simulink model "compute_next_state_2019a"  (R2019a)
settings: Solver=FixedStepAuto  StartTime=0.0  StopTime=10.0  FixedStep=0.5  RelTol=1e-3
settings Model: Creator=Julius  LastModifiedBy=Julius
settings DebuggingCC: SFMachineParentedDataDiag=error

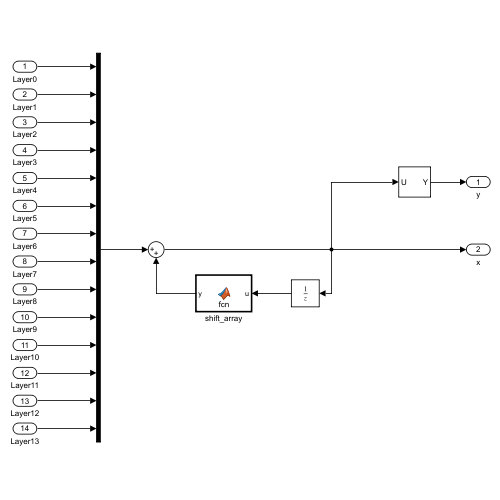
[thumbnail: Simulink's stored preview of the top-level diagram]
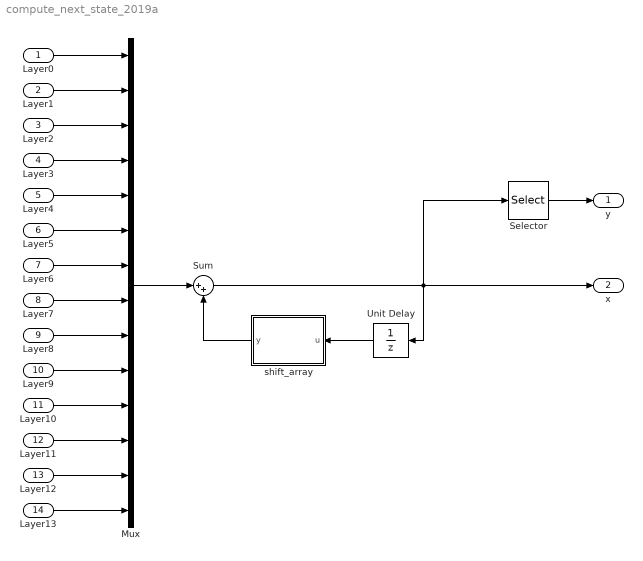
== system compute_next_state_2019a ==
  Layer0 : Inport  OutDataTypeStr=double  PortDimensions=1
  Layer1 : Inport  Port=2  OutDataTypeStr=double  PortDimensions=1
  Layer2 : Inport  Port=3  OutDataTypeStr=double  PortDimensions=1
  Layer3 : Inport  Port=4  OutDataTypeStr=double  PortDimensions=1
  Layer4 : Inport  Port=5  OutDataTypeStr=double  PortDimensions=1
  Layer5 : Inport  Port=6  OutDataTypeStr=double  PortDimensions=1
  Layer6 : Inport  Port=7  OutDataTypeStr=double  PortDimensions=1
  Layer7 : Inport  Port=8  OutDataTypeStr=double  PortDimensions=1
  Layer8 : Inport  Port=9  OutDataTypeStr=double  PortDimensions=1
  Layer9 : Inport  Port=10  OutDataTypeStr=double  PortDimensions=1
  Layer10 : Inport  Port=11  OutDataTypeStr=double  PortDimensions=1
  Layer11 : Inport  Port=12  OutDataTypeStr=double  PortDimensions=1
  Layer12 : Inport  Port=13  OutDataTypeStr=double  PortDimensions=1
  Layer13 : Inport  Port=14  OutDataTypeStr=double  PortDimensions=1
  Mux : Mux  Inputs=14
  Selector : Selector  IndexMode=Zero-based  InputPortWidth=14  IndexOptions=Index vector (dialog)  Indices=[1 1]  OutputSizes=1
  Sum : Sum  Inputs=|++
  Unit Delay : UnitDelay  InitialCondition=zeros(14, 1)  SampleTime=-1  HasFrameUpgradeWarning=on
  shift_array : MATLAB Function  TreatAsAtomicUnit=on
  y : Outport
  x : Outport  Port=2  PortDimensions=14
  wires:
  Mux/1 -> Sum/1
  Unit Delay/1 -> shift_array/1(u)
  shift_array/1(y) -> Sum/2
  Layer3/1 -> Mux/4
  Layer4/1 -> Mux/5
  Layer12/1 -> Mux/13
  Layer8/1 -> Mux/9
  Layer0/1 -> Mux/1
  Layer13/1 -> Mux/14
  Layer1/1 -> Mux/2
  Layer11/1 -> Mux/12
  Layer5/1 -> Mux/6
  Layer6/1 -> Mux/7
  Layer10/1 -> Mux/11
  Layer2/1 -> Mux/3
  Layer9/1 -> Mux/10
  Layer7/1 -> Mux/8
  Selector/1 -> y/1
  Sum/1 -> x/1, Selector/1, Unit Delay/1

== matlab function compute_next_state_2019a/shift_array ==
  data: u input; y output
function y = fcn(u)
y = [u(2:end, 1); 0];
